simulink model "bicyclops"  (R2018b)
settings: Solver=VariableStepAuto  StartTime=0.0  StopTime=tmax  MaxStep=dt  RelTol=1e-3
InitFcn:
  | m = 1452; % Mass of Vehicle (kg)
  | J = 2200; % Moment of Inertia (kg-m^2)
  | Jx = 510; % Roll Moment of Inertia (kg-m^2)
  | L = 2.7; % Wheel base of Vehicle (m)
  | vx = 28; % Longitudinal Velocity (m/s)== 100kph
  | Cf = 50000; % Conering Coefficient of Front Tire (N/rad)
  | tmax = 10;
  | dt = 0.001;
  | 
undefined symbols (not defined in the file): init, sigbuilder_block
settings Model: Creator=zac  LastModifiedBy=GangC
settings DataIOCC: SaveFormat=Array  SaveOutput=off  SignalLogging=off  DSMLogging=off  SaveTime=off  SignalLoggingName=datasave
settings DebuggingCC: LibraryContextMissingDiagnostic=none
settings SFSimCC: SimUseLocalCustomCode=off
settings RTWCC: RTWUseLocalCustomCode=off
settings CodeAppCC: StateflowObjectComments=on

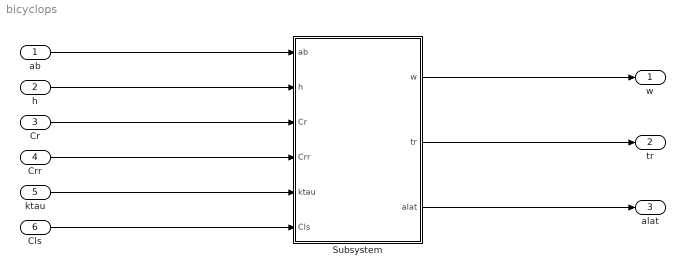
== system bicyclops ==
  ab : Inport
  h : Inport  Port=2
  Cr : Inport  Port=3
  Crr : Inport  Port=4
  ktau : Inport  Port=5
  Cls : Inport  Port=6
  Subsystem : Subsystem
  w : Outport
  tr : Outport  Port=2
  alat : Outport  Port=3
  wires:
  ab/1 -> Subsystem/1(ab)
  h/1 -> Subsystem/2(h)
  Cr/1 -> Subsystem/3(Cr)
  Crr/1 -> Subsystem/4(Crr)
  ktau/1 -> Subsystem/5(ktau)
  Cls/1 -> Subsystem/6(Cls)
  Subsystem/1(w) -> w/1
  Subsystem/2(tr) -> tr/1
  Subsystem/3(alat) -> alat/1

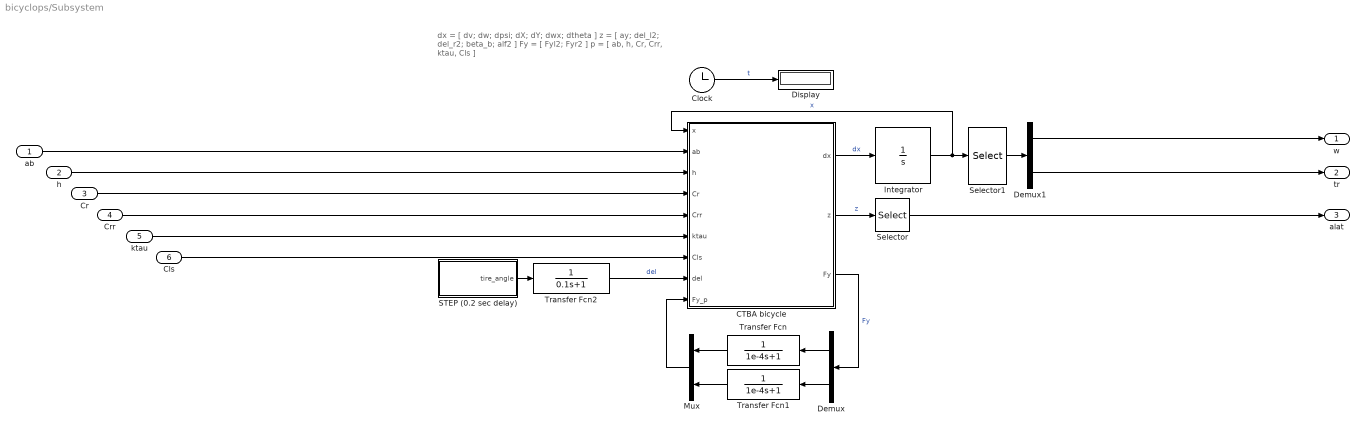
== system bicyclops/Subsystem ==
  note: dx = [ dv; dw; dpsi; dX; dY; dwx; dtheta ]
      | z = [ ay; del_l2; del_r2; beta_b; alf2 ]
      | Fy = [ Fyl2; Fyr2 ]
      | p = [ ab, h, Cr, Crr, ktau, Cls ]
  ab : Inport
  h : Inport  Port=2
  Cr : Inport  Port=3
  Crr : Inport  Port=4
  ktau : Inport  Port=5
  Cls : Inport  Port=6
  CTBA bicycle : MATLAB Function  TreatAsAtomicUnit=on
  Clock : Clock
  Demux : Demux  Outputs=2
  Demux1 : Demux  Outputs=2
  Display : Display
  Integrator : Integrator  InitialCondition=init
  Mux : Mux  Inputs=2
  STEP (0.2 sec delay) : Subsystem  Tag=STV Subsys  LoadFcn=sigbuilder_block('load');  StartFcn=sigbuilder_block('start');  StopFcn=sigbuilder_block('stop');  ClipboardFcn=sigbuilder_block('clipboard');  mask(Sigbuilder block){tuvar=[0:10]}
      mask help: Simulink:masks:SigbuilderBlock_MD
      mask init:
      | if ~strcmp(get_param(bdroot(gcbh),'SimulationStatus'),'stopped') tuvar = sigbuilder_block('maskInit'); end
      settings: CopyFcn=sigbuilder_block('copy');  DeleteFcn=sigbuilder_block('delete');  ModelCloseFcn=sigbuilder_block('modelClose');  PreSaveFcn=sigbuilder_block('preSave');  PauseFcn=sigbuilder_block('pause');  ContinueFcn=sigbuilder_block('continue');  NameChangeFcn=sigbuilder_block('namechange');  OpenFcn=sigbuilder_block('open',[567 140.25 550.5 399.75 ]);  CloseFcn=sigbuilder_block('close');
      mask Display: plot(0, 0, 100, 100,[2, 2, 32, 32, 2], [68, 8, 8, 68, 68],[32, 2], [38, 38], [32, 19, 2],[53, 60, 44], [32, 17, 17, 2],[16, 16, 31, 31]);txt = getActiveGroup(gcbh);text(2, 100, txt,'verticalAlignment', 'top');
  Selector : Selector  InputPortWidth=5  IndexOptions=Index vector (dialog)  Indices=1  OutputSizes=1
  Selector1 : Selector  InputPortWidth=7  IndexOptions=Index vector (dialog)  Indices=[2 7]  OutputSizes=1
  Transfer Fcn : TransferFcn  Denominator=[1e-4 1]
  Transfer Fcn1 : TransferFcn  Denominator=[1e-4 1]
  Transfer Fcn2 : TransferFcn  Denominator=[0.1 1]
  w : Outport
  tr : Outport  Port=2
  alat : Outport  Port=3
  wires:
  Mux/1 -> CTBA bicycle/9(Fy_p)
  Transfer Fcn1/1 -> Mux/2
  STEP (0.2 sec delay)/1(tire_angle) -> Transfer Fcn2/1
  CTBA bicycle/1(dx) -> Integrator/1  "dx"
  Demux/2 -> Transfer Fcn1/1
  Integrator/1 -> CTBA bicycle/1(x), Selector1/1  "x"
  Transfer Fcn2/1 -> CTBA bicycle/8(del)  "del"
  CTBA bicycle/3(Fy) -> Demux/1  "Fy"
  CTBA bicycle/2(z) -> Selector/1  "z"
  Selector1/1 -> Demux1/1
  Demux/1 -> Transfer Fcn/1
  Clock/1 -> Display/1  "t"
  Transfer Fcn/1 -> Mux/1
  ktau/1 -> CTBA bicycle/6(ktau)
  ab/1 -> CTBA bicycle/2(ab)
  Crr/1 -> CTBA bicycle/5(Crr)
  Cr/1 -> CTBA bicycle/4(Cr)
  h/1 -> CTBA bicycle/3(h)
  Selector/1 -> alat/1
  Cls/1 -> CTBA bicycle/7(Cls)
  Demux1/2 -> tr/1
  Demux1/1 -> w/1

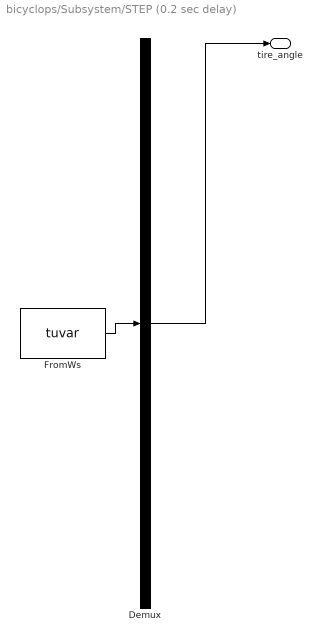
== system bicyclops/Subsystem/STEP (0.2 sec delay) ==
  Demux : Demux  Tag=STV Demux  Outputs=1
  FromWs : FromWorkspace  Tag=STV FromWs  VariableName=tuvar  SampleTime=0
      SigBuilderData=|
      | common.afterFinalStr = 'Extrapolate'
      | common.sampleTime = 0
      | dataSet.timeRange = [0 10]
      | dataSet.name = 'steering'
      | sbobj.Groups.Name = 'steering'
      | sbobj.Groups.Signals.Name = 'tire_angle'
      | sbobj.Groups.Signals.XData = [0 2 2.2 10]
      | sbobj.Groups.Signals.YData = [0 0 0.0349065850399 0.0349065850399]
  tire_angle : Outport  Tag=STV Outport
  wires:
  Demux/1 -> tire_angle/1
  FromWs/1 -> Demux/1

== matlab function bicyclops/Subsystem/CTBA bicycle ==
  data: x input; ab input; h input; Cr input; Crr input; ktau input; Cls input; dx output; del input; Fy_p input; z output; Fy output; m parameter; J parameter; Jx parameter; Cf parameter; vx parameter; L parameter
function [dx,z,Fy] = ctbabike(x, ab, h, Cr, Crr, ktau, Cls, del, Fy_p, ...
    m, J, Jx, Cf, vx, L)

% m, J, Jx, a, b, h, Cf, Cr, Crr, ktau, Cls, vx
% p to change: ab, h, Cr, Crr, ktau, Cls
b = L/(1 + ab);
a = L - b;
% Unpack states
v = x(1);
w = x(2);
psi = x(3);
% X = x(4);
% Y = x(5);
wx = x(6);
theta = x(7);
% Unpack previous tire forces
Fyl2_p = Fy_p(1);
Fyr2_p = Fy_p(2);

% Rear Steer Angle using the previous tire force
del_l2 = Crr*theta + Cls*(Fyl2_p+Fyr2_p); % Rear-left steer angle
del_r2 = Crr*theta + Cls*(Fyl2_p+Fyr2_p); % Rear-right steer angle

% Front and rear slip angles
alf1 = del - (v + a*w)/vx;
alf2 = -(v - b*w)/vx;

% % Equivalent rear axle slip angle
% D = (2*Cr*Crr*h - ktau + 2*Cls*Cr*ktau);
% beta1 = -2*Cf*Crr*h/D;
% beta2 = -ktau/D;
% alf2_mod = beta1*alf1 + beta2*alf2;

% Front tire forces
% - Assume no suspension effects
Fyl1 = Cf*alf1;
Fyr1 = Cf*alf1;

% Rear lateral tire forces
% Fyl2 = Cr*alf2_mod;
% Fyr2 = Cr*alf2_mod;
Fyl2 = Cr*(alf2 + del_l2);
Fyr2 = Cr*(alf2 + del_r2);

% Total lateral tire force
Fy_all = Fyl1 + Fyr1 + Fyl2 + Fyr2;

% Equations of motion
dv = 1/m*Fy_all - w*vx;
dw = 1/J*(a*(Fyl1 + Fyr1) - b*(Fyl2 + Fyr2));
dpsi = w;
dX = vx*cos(psi) - v*sin(psi);
dY = vx*sin(psi) + v*cos(psi);
dwx = 1/Jx*(-ktau*theta + Fy_all*h - 4*(1.5/2)^2*2.9400e+03*wx); %-4*(1.5/2)^2*2.9400e+03*wx
dtheta = wx;

% Additional outputs
ay = dv + vx*w; % Lateral acceleration
% del_l2 = Crr*Fy_all*h/ktau + Cls*(Fyl2 + Fyr2); % Rear-left steer angle
% del_r2 = Crr*Fy_all*h/ktau + Cls*(Fyl2 + Fyr2); % Rear-right steer angle
beta_b = atan(v/vx); % Body slip angle

% Pack output vectors
dx = [dv; dw; dpsi; dX; dY; dwx; dtheta];
z = [ay; del_l2; del_r2; beta_b; alf2];
Fy = [Fyl2;Fyr2];
